simulink model "simulation23"  (R2015b)
settings: Solver=VariableStepAuto  StartTime=0.0  StopTime=1500  RelTol=1e-3
values from neighbouring files (symbols this model uses):
  g = 9.81    [constantsForControlGains.m]
  Kd_phi = (2*zeta_phi*omega_n_phi - a_phi_1)/a_phi_2    [controlGains.m]
  Ki_kji = omega_n_kji^2 * Va/g    [controlGains.m]
  Ki_phi = 0    [controlGains.m]
  Kp_kji = 2*zeta_kji*omega_n_kji*Va/g    [controlGains.m]
  Kp_phi = (delta_a_max/e_phi_max) * sign(a_phi_2)    [controlGains.m]
  step_course_hold = 25    [stepsForCourseHoldAndManeuvers.m]
  step_course_hold_start_time = 200    [stepsForCourseHoldAndManeuvers.m]
  step_manuever1 = 20    [stepsForCourseHoldAndManeuvers.m]
  step_manuever1_start_time = 200    [stepsForCourseHoldAndManeuvers.m]
  step_manuever2 = 60    [stepsForCourseHoldAndManeuvers.m]
  step_manuever2_start_time = 400    [stepsForCourseHoldAndManeuvers.m]
  step_manuever3 = 70    [stepsForCourseHoldAndManeuvers.m]
  step_manuever3_start_time = 600    [stepsForCourseHoldAndManeuvers.m]
  step_manuever4 = -50    [stepsForCourseHoldAndManeuvers.m]
  step_manuever4_start_time = 800    [stepsForCourseHoldAndManeuvers.m]
  step_manuever5 = -80    [stepsForCourseHoldAndManeuvers.m]
  step_manuever5_start_time = 1000    [stepsForCourseHoldAndManeuvers.m]
  step_manuever6 = -60    [stepsForCourseHoldAndManeuvers.m]
  step_manuever6_start_time = 1200    [stepsForCourseHoldAndManeuvers.m]
  T = 20    [stepsForCourseHoldAndManeuvers.m]
  Va = 552/3.6    (= 153.333333333)    [constantsForControlGains.m]
undefined symbols (not defined in the file or in its folder): A, B, C
libraries: simulink_extras x6
settings Model: Creator=ShivJeet  LastModifiedBy=ShivJeet

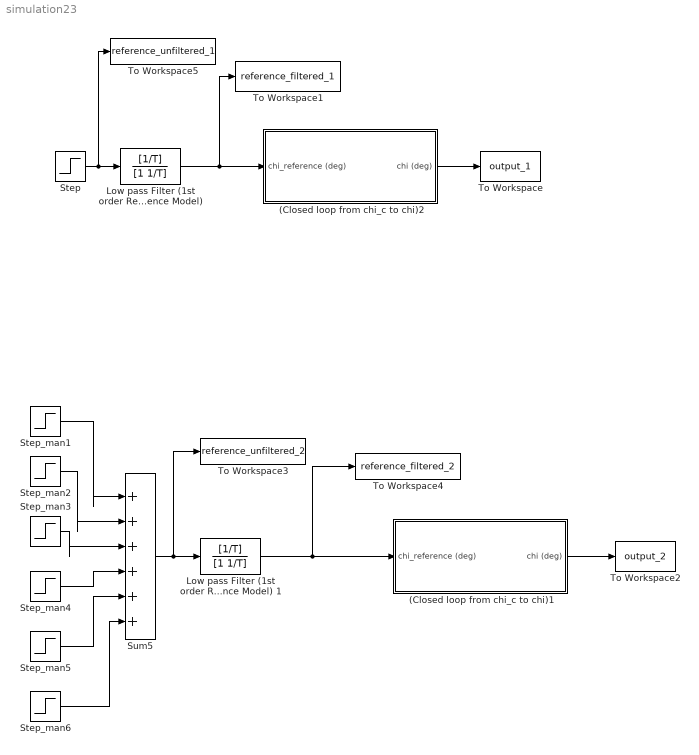
== system simulation23 ==
  (Closed loop from chi_c to chi)1 : Subsystem
  (Closed loop from chi_c to chi)2 : Subsystem
  "Low pass Filter (1st order Reference Model) " : TransferFcn  Numerator=[1/T]  Denominator=[1 1/T]
  Low pass Filter (1st order Reference Model) 1 : TransferFcn  Numerator=[1/T]  Denominator=[1 1/T]
  Step : Step  Time=step_course_hold_start_time  After=step_course_hold  SampleTime=0
  Step_man1 : Step  Time=step_manuever1_start_time  After=step_manuever1  SampleTime=0
  Step_man2 : Step  Time=step_manuever2_start_time  After=step_manuever2  SampleTime=0
  Step_man3 : Step  Time=step_manuever3_start_time  After=step_manuever3  SampleTime=0
  Step_man4 : Step  Time=step_manuever4_start_time  After=step_manuever4  SampleTime=0
  Step_man5 : Step  Time=step_manuever5_start_time  After=step_manuever5  SampleTime=0
  Step_man6 : Step  Time=step_manuever6_start_time  After=step_manuever6  SampleTime=0
  Sum5 : Sum  Inputs=|++++++
  To Workspace : ToWorkspace  VariableName=output_1  SaveFormat=Timeseries  SampleTime=-1
  To Workspace1 : ToWorkspace  VariableName=reference_filtered_1  SaveFormat=Timeseries  SampleTime=-1
  To Workspace2 : ToWorkspace  VariableName=output_2  SaveFormat=Timeseries  SampleTime=-1
  To Workspace3 : ToWorkspace  VariableName=reference_unfiltered_2  SaveFormat=Timeseries  SampleTime=-1
  To Workspace4 : ToWorkspace  VariableName=reference_filtered_2  SaveFormat=Timeseries  SampleTime=-1
  To Workspace5 : ToWorkspace  VariableName=reference_unfiltered_1  SaveFormat=Timeseries  SampleTime=-1
  wires:
  Step/1 -> To Workspace5/1, "Low pass Filter (1st order Reference Model) "/1
  (Closed loop from chi_c to chi)1/1(chi (deg)) -> To Workspace2/1
  Sum5/1 -> To Workspace3/1, Low pass Filter (1st order Reference Model) 1/1
  Step_man1/1 -> Sum5/1
  Step_man2/1 -> Sum5/2
  Step_man3/1 -> Sum5/3
  Step_man4/1 -> Sum5/4
  Step_man5/1 -> Sum5/5
  Step_man6/1 -> Sum5/6
  (Closed loop from chi_c to chi)2/1(chi (deg)) -> To Workspace/1
  "Low pass Filter (1st order Reference Model) "/1 -> (Closed loop from chi_c to chi)2/1(chi_reference (deg)), To Workspace1/1
  Low pass Filter (1st order Reference Model) 1/1 -> To Workspace4/1, (Closed loop from chi_c to chi)1/1(chi_reference (deg))

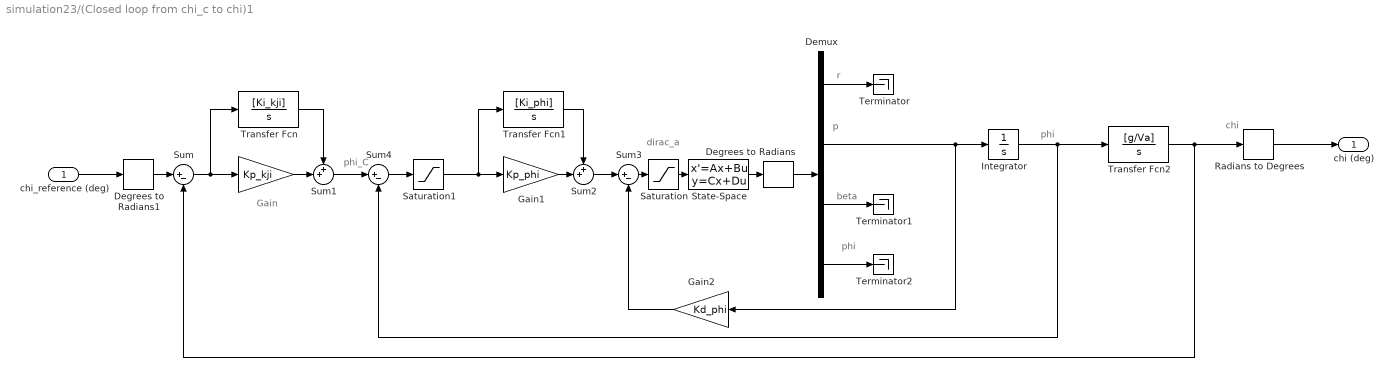
== system simulation23/(Closed loop from chi_c to chi)1 ==
  note: Gain
  note: dirac_a
  note: phi
  note: beta
  note: r
  note: phi_C
  note: chi
  note: phi
  note: p
  chi_reference (deg) : Inport
  " " : Gain  Gain=Kp_kji
  Degrees to Radians : simulink_extras/Transformations/Degrees to Radians
  Degrees to Radians1 : simulink_extras/Transformations/Degrees to Radians
  Demux : Demux
  Gain1 : Gain  Gain=Kp_phi
  Gain2 : Gain  Gain=Kd_phi
  Integrator : Integrator
  Radians to Degrees : simulink_extras/Transformations/Radians to Degrees
  Saturation : Saturate  UpperLimit=45 * pi/180  LowerLimit=- 45 * pi/180
  Saturation1 : Saturate  UpperLimit=15 * pi/180  LowerLimit=- 15 * pi/180
  State-Space : StateSpace  A=A  B=B(:,1)  C=C  D=[0; 0; 0; 0;]  X0=0
  Sum : Sum  Inputs=|+-
  Sum1 : Sum  Inputs=++|
  Sum2 : Sum  Inputs=++|
  Sum3 : Sum  Inputs=|+-
  Sum4 : Sum  Inputs=|+-
  Terminator : Terminator
  Terminator1 : Terminator
  Terminator2 : Terminator
  Transfer Fcn : TransferFcn  Numerator=[Ki_kji]  Denominator=[1 0]
  Transfer Fcn1 : TransferFcn  Numerator=[Ki_phi]  Denominator=[1 0]
  Transfer Fcn2 : TransferFcn  Numerator=[g/Va]  Denominator=[1 0]
  chi (deg) : Outport
  wires:
  chi_reference (deg)/1 -> Degrees to Radians1/1
  Demux/1 -> Terminator/1
  Radians to Degrees/1 -> chi (deg)/1
  Demux/4 -> Terminator2/1
  Degrees to Radians/1 -> Demux/1
  Sum/1 -> Transfer Fcn/1, " "/1
  Gain1/1 -> Sum2/2
  State-Space/1 -> Degrees to Radians/1
  Demux/2 -> Integrator/1, Gain2/1
  Degrees to Radians1/1 -> Sum/1
  Sum2/1 -> Sum3/1
  Sum1/1 -> Sum4/1
  Sum4/1 -> Saturation1/1
  Gain2/1 -> Sum3/2
  Transfer Fcn2/1 -> Radians to Degrees/1, Sum/2
  " "/1 -> Sum1/2
  Transfer Fcn1/1 -> Sum2/1
  Integrator/1 -> Transfer Fcn2/1, Sum4/2
  Transfer Fcn/1 -> Sum1/1
  Demux/3 -> Terminator1/1
  Sum3/1 -> Saturation/1
  Saturation/1 -> State-Space/1
  Saturation1/1 -> Transfer Fcn1/1, Gain1/1

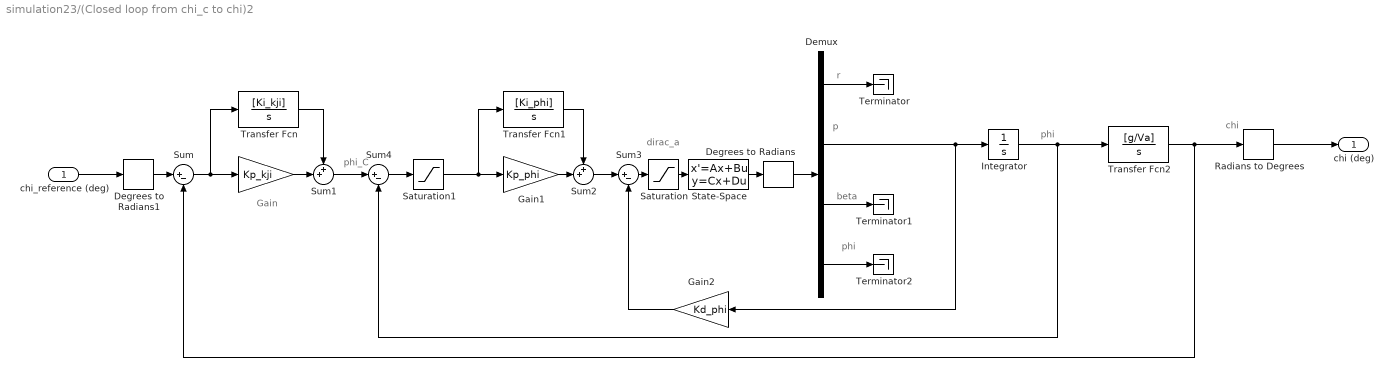
== system simulation23/(Closed loop from chi_c to chi)2 ==
  note: Gain
  note: dirac_a
  note: phi
  note: beta
  note: r
  note: phi_C
  note: chi
  note: phi
  note: p
  chi_reference (deg) : Inport
  " " : Gain  Gain=Kp_kji
  Degrees to Radians : simulink_extras/Transformations/Degrees to Radians
  Degrees to Radians1 : simulink_extras/Transformations/Degrees to Radians
  Demux : Demux
  Gain1 : Gain  Gain=Kp_phi
  Gain2 : Gain  Gain=Kd_phi
  Integrator : Integrator
  Radians to Degrees : simulink_extras/Transformations/Radians to Degrees
  Saturation : Saturate  UpperLimit=45 * pi/180  LowerLimit=- 45 * pi/180
  Saturation1 : Saturate  UpperLimit=15 * pi/180  LowerLimit=- 15 * pi/180
  State-Space : StateSpace  A=A  B=B(:,1)  C=C  D=[0; 0; 0; 0;]  X0=0
  Sum : Sum  Inputs=|+-
  Sum1 : Sum  Inputs=++|
  Sum2 : Sum  Inputs=++|
  Sum3 : Sum  Inputs=|+-
  Sum4 : Sum  Inputs=|+-
  Terminator : Terminator
  Terminator1 : Terminator
  Terminator2 : Terminator
  Transfer Fcn : TransferFcn  Numerator=[Ki_kji]  Denominator=[1 0]
  Transfer Fcn1 : TransferFcn  Numerator=[Ki_phi]  Denominator=[1 0]
  Transfer Fcn2 : TransferFcn  Numerator=[g/Va]  Denominator=[1 0]
  chi (deg) : Outport
  wires:
  chi_reference (deg)/1 -> Degrees to Radians1/1
  Demux/1 -> Terminator/1
  Radians to Degrees/1 -> chi (deg)/1
  Demux/4 -> Terminator2/1
  Degrees to Radians/1 -> Demux/1
  Sum/1 -> Transfer Fcn/1, " "/1
  Gain1/1 -> Sum2/2
  State-Space/1 -> Degrees to Radians/1
  Demux/2 -> Integrator/1, Gain2/1
  Degrees to Radians1/1 -> Sum/1
  Sum2/1 -> Sum3/1
  Sum1/1 -> Sum4/1
  Sum4/1 -> Saturation1/1
  Gain2/1 -> Sum3/2
  Transfer Fcn2/1 -> Radians to Degrees/1, Sum/2
  " "/1 -> Sum1/2
  Transfer Fcn1/1 -> Sum2/1
  Integrator/1 -> Transfer Fcn2/1, Sum4/2
  Transfer Fcn/1 -> Sum1/1
  Demux/3 -> Terminator1/1
  Sum3/1 -> Saturation/1
  Saturation/1 -> State-Space/1
  Saturation1/1 -> Transfer Fcn1/1, Gain1/1
